simulink model "Reservoir_mdl"  (R2017b)
settings: Solver=VariableStepAuto  StartTime=0.0  StopTime=200  MaxStep=1e-3  MinStep=1e-4  RelTol=1e-3
values from neighbouring files (symbols this model uses):
  A = [-0.2415 0.2415 0;0.2415 -0.4244 0.1566;0 0.1566 -0.1865]    [Reservoir.m]
  A11 = [A(1,1) A(1,2);A(2,1) A(2,2)]    [Reservoir.m]
  A12 = [A(1,3);A(2,3)]    [Reservoir.m]
  A21 = [A(3,1) A(3,2)]    [Reservoir.m]
  A22 = A(3,3)    [Reservoir.m]
  B = [795.7747;0;0]    [Reservoir.m]
  B1 = B(1:2)    [Reservoir.m]
  B2 = B(2:end)    [Reservoir.m]
  C = [0 0 1]    [Reservoir.m]
  Ka = acker(Aa,Ba,Pa)    [Reservoir.m]
  L2 = L(1:2)    [Reservoir.m]
settings Model: Creator=info  LastModifiedBy=info

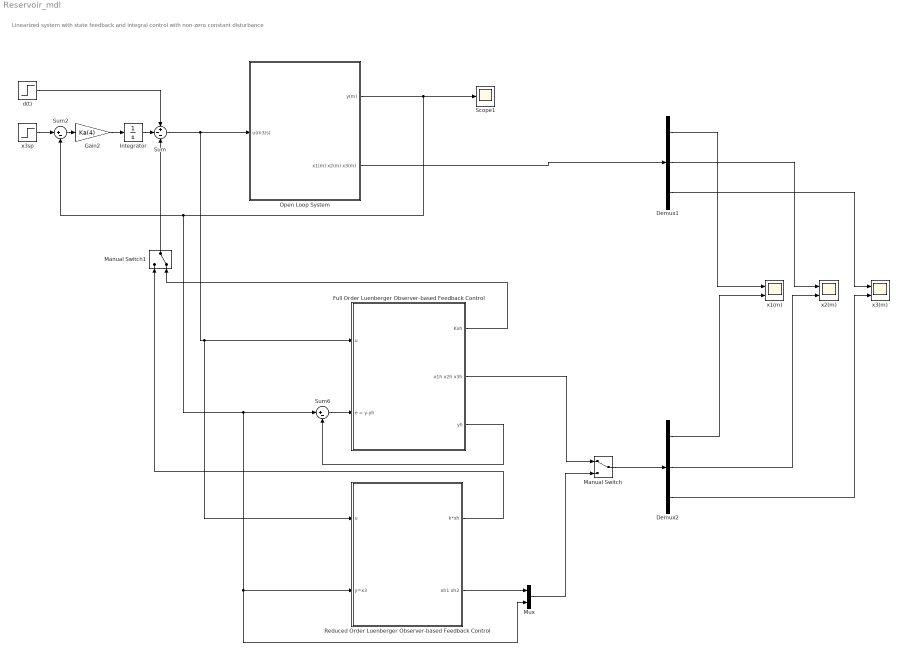
== system Reservoir_mdl ==
  note: Linearized system with state feedback and integral control
      |                                                                                                 with non-zero constant disturbance
  Demux1 : Demux  Outputs=3
  Demux2 : Demux  Outputs=3
  Full Order Luenberger Observer-based Feedback Control : Subsystem
  Gain2 : Gain  Gain=Ka(4)
  Integrator : Integrator
  Manual Switch : ManualSwitch
  Manual Switch1 : ManualSwitch  CurrentSetting=0
  Mux : Mux  Inputs=2
  Open Loop System : Subsystem
  Reduced Order Luenberger Observer-based Feedback Control : Subsystem
  Scope1 : Scope
  Sum : Sum  Inputs=+--
  Sum2 : Sum  Inputs=|+-
  Sum6 : Sum  Inputs=|+-
  d(t) : Step  Time=75  After=0  SampleTime=0
  x1(m) : Scope  NumInputPorts=2
  x2(m) : Scope  NumInputPorts=2
  x3(m) : Scope  NumInputPorts=2
  x3sp : Step  Time=0  After=0.25  SampleTime=0
  wires:
  x3sp/1 -> Sum2/1
  Sum2/1 -> Gain2/1
  Gain2/1 -> Integrator/1
  Integrator/1 -> Sum/2
  d(t)/1 -> Sum/1
  Sum6/1 -> Full Order Luenberger Observer-based Feedback Control/2(e = y-yh)
  Full Order Luenberger Observer-based Feedback Control/3(yh) -> Sum6/2
  Sum/1 -> Open Loop System/1(u(m3/s)), Full Order Luenberger Observer-based Feedback Control/1(u), Reduced Order Luenberger Observer-based Feedback Control/1(u)
  Open Loop System/1(y(m)) -> Sum6/1, Mux/2, Reduced Order Luenberger Observer-based Feedback Control/2(y=x3), Sum2/2, Scope1/1
  Open Loop System/2(x1(m) x2(m) x3(m)) -> Demux1/1
  Demux2/1 -> x1(m)/2
  Demux1/1 -> x1(m)/1
  Demux1/2 -> x2(m)/1
  Demux2/2 -> x2(m)/2
  Demux2/3 -> x3(m)/2
  Demux1/3 -> x3(m)/1
  Manual Switch/1 -> Demux2/1
  Full Order Luenberger Observer-based Feedback Control/2(x1h x2h x3h) -> Manual Switch/1
  Mux/1 -> Manual Switch/2
  Reduced Order Luenberger Observer-based Feedback Control/2(xh1 xh2) -> Mux/1
  Full Order Luenberger Observer-based Feedback Control/1(Kxh) -> Manual Switch1/2
  Manual Switch1/1 -> Sum/3
  Reduced Order Luenberger Observer-based Feedback Control/1(k*xh) -> Manual Switch1/1

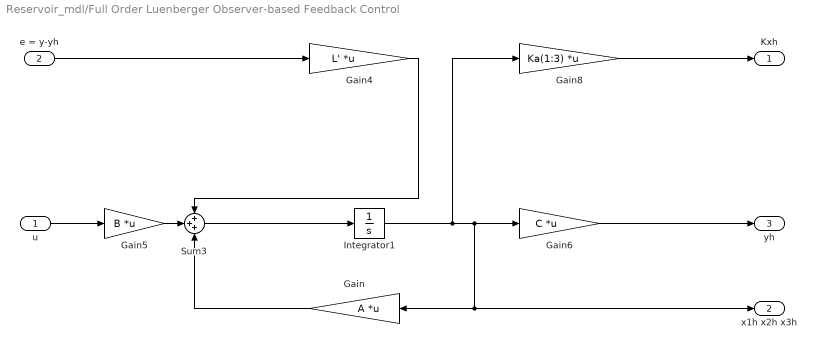
== system Reservoir_mdl/Full Order Luenberger Observer-based Feedback Control ==
  u : Inport
  e = y-yh : Inport  Port=2
  Gain : Gain  Gain=A  Multiplication=Matrix(K*u) (u vector)
  Gain4 : Gain  Gain=L'  Multiplication=Matrix(K*u) (u vector)
  Gain5 : Gain  Gain=B  Multiplication=Matrix(K*u) (u vector)
  Gain6 : Gain  Gain=C  Multiplication=Matrix(K*u) (u vector)
  Gain8 : Gain  Gain=Ka(1:3)  Multiplication=Matrix(K*u) (u vector)
  Integrator1 : Integrator  InitialCondition=[1;1;2]
  Sum3 : Sum  Inputs=+++
  Kxh : Outport
  x1h x2h x3h : Outport  Port=2
  yh : Outport  Port=3
  wires:
  Gain4/1 -> Sum3/1
  Integrator1/1 -> Gain6/1, x1h x2h x3h/1, Gain/1, Gain8/1
  u/1 -> Gain5/1
  Gain8/1 -> Kxh/1
  Sum3/1 -> Integrator1/1
  Gain5/1 -> Sum3/2
  Gain/1 -> Sum3/3
  Gain6/1 -> yh/1
  e = y-yh/1 -> Gain4/1

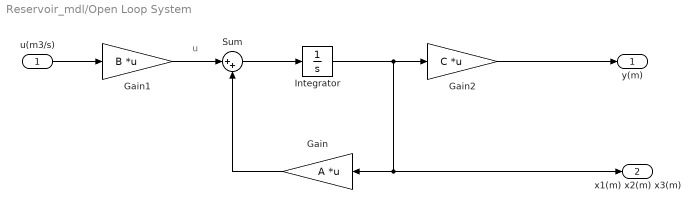
== system Reservoir_mdl/Open Loop System ==
  note: u
  u(m3/s) : Inport
  Gain : Gain  Gain=A  Multiplication=Matrix(K*u) (u vector)
  Gain1 : Gain  Gain=B  Multiplication=Matrix(K*u) (u vector)
  Gain2 : Gain  Gain=C  Multiplication=Matrix(K*u) (u vector)
  Integrator : Integrator
  Sum : Sum  Inputs=|++
  y(m) : Outport
  x1(m) x2(m) x3(m) : Outport  Port=2
  wires:
  Integrator/1 -> Gain2/1, Gain/1, x1(m) x2(m) x3(m)/1
  Gain2/1 -> y(m)/1
  Sum/1 -> Integrator/1
  Gain1/1 -> Sum/1
  Gain/1 -> Sum/2
  u(m3/s)/1 -> Gain1/1

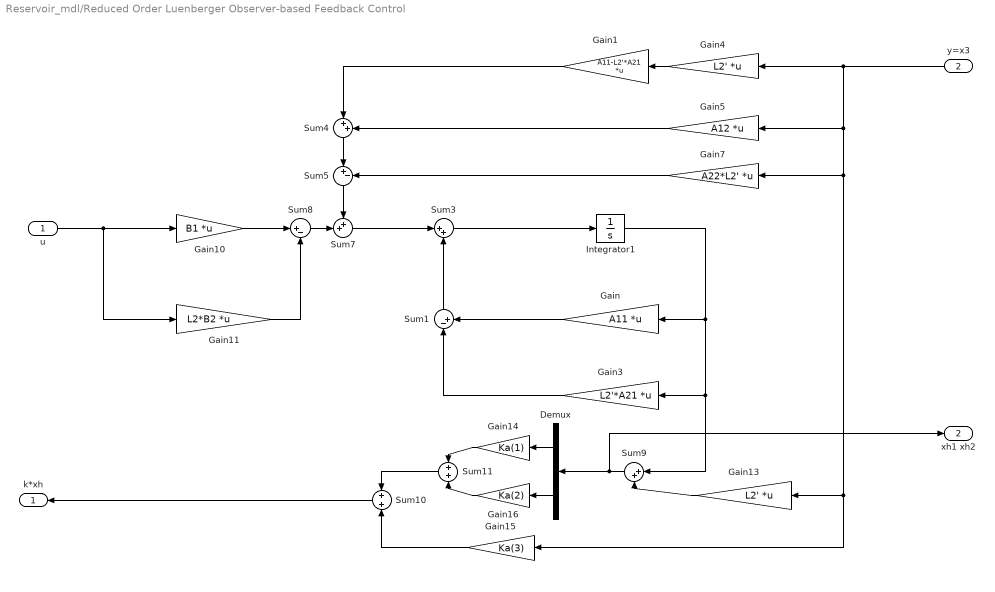
== system Reservoir_mdl/Reduced Order Luenberger Observer-based Feedback Control ==
  u : Inport
  y=x3 : Inport  Port=2
  Demux : Demux  Outputs=2
  Gain : Gain  Gain=A11  Multiplication=Matrix(K*u) (u vector)
  Gain1 : Gain  Gain=A11-L2'*A21  Multiplication=Matrix(K*u) (u vector)
  Gain10 : Gain  Gain=B1  Multiplication=Matrix(K*u) (u vector)
  Gain11 : Gain  Gain=L2*B2  Multiplication=Matrix(K*u) (u vector)
  Gain13 : Gain  Gain=L2'  Multiplication=Matrix(K*u) (u vector)
  Gain14 : Gain  Gain=Ka(1)
  Gain15 : Gain  Gain=Ka(3)
  Gain16 : Gain  Gain=Ka(2)
  Gain3 : Gain  Gain=L2'*A21  Multiplication=Matrix(K*u) (u vector)
  Gain4 : Gain  Gain=L2'  Multiplication=Matrix(K*u) (u vector)
  Gain5 : Gain  Gain=A12  Multiplication=Matrix(K*u) (u vector)
  Gain7 : Gain  Gain=A22*L2'  Multiplication=Matrix(K*u) (u vector)
  Integrator1 : Integrator  InitialCondition=[1;0.5]
  Sum1 : Sum  Inputs=|-+
  Sum10 : Sum
  Sum11 : Sum
  Sum3 : Sum  Inputs=|++
  Sum4 : Sum  Inputs=|++
  Sum5 : Sum  Inputs=|+-
  Sum7 : Sum  Inputs=++|
  Sum8 : Sum  Inputs=|+-
  Sum9 : Sum  Inputs=|++
  k*xh : Outport
  xh1 xh2 : Outport  Port=2
  wires:
  Demux/1 -> Gain14/1
  Gain13/1 -> Sum9/2
  Sum10/1 -> k*xh/1
  Gain/1 -> Sum1/2
  Sum4/1 -> Sum5/1
  Gain5/1 -> Sum4/2
  Gain1/1 -> Sum4/1
  Gain7/1 -> Sum5/2
  Sum5/1 -> Sum7/1
  Gain15/1 -> Sum10/2
  Sum11/1 -> Sum10/1
  Gain3/1 -> Sum1/1
  Gain16/1 -> Sum11/2
  Demux/2 -> Gain16/1
  Gain4/1 -> Gain1/1
  Sum7/1 -> Sum3/1
  Sum8/1 -> Sum7/2
  Gain14/1 -> Sum11/1
  Sum3/1 -> Integrator1/1
  Sum1/1 -> Sum3/2
  Gain11/1 -> Sum8/2
  Gain10/1 -> Sum8/1
  Integrator1/1 -> Sum9/1, Gain3/1, Gain/1
  Sum9/1 -> xh1 xh2/1, Demux/1
  u/1 -> Gain11/1, Gain10/1
  y=x3/1 -> Gain4/1, Gain5/1, Gain15/1, Gain13/1, Gain7/1
